simulink model "math_red"  (Simulink 6.6)
settings: Solver=FixedStepDiscrete  StartTime=0.0  StopTime=10.0  FixedStep=1  RelTol=1e-3
settings Model: Creator=ksmyth  LastModifiedBy=Nyenyec

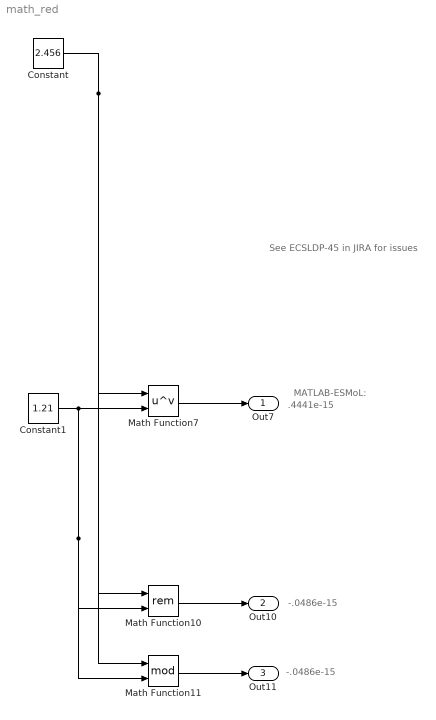
== system math_red ==
  note: MATLAB-ESMoL:
  note: .4441e-15
  note: -.0486e-15
  note: -.0486e-15
  note: See ECSLDP-45 in JIRA for issues
  Constant : Constant  Value=2.456
  Constant1 : Constant  Value=1.21
  Math Function10 : Math  Operator=rem  SaturateOnIntegerOverflow=on
  Math Function11 : Math  Operator=mod  SaturateOnIntegerOverflow=on
  Math Function7 : Math  Operator=pow  SaturateOnIntegerOverflow=on
  Out7 : Outport
  Out10 : Outport  Port=2
  Out11 : Outport  Port=3
  wires:
  Constant/1 -> Math Function10/1, Math Function11/1, Math Function7/1
  Math Function7/1 -> Out7/1
  Constant1/1 -> Math Function7/2, Math Function11/2, Math Function10/2
  Math Function10/1 -> Out10/1
  Math Function11/1 -> Out11/1
